simulink library "csbenchlab_sys"  (R2024a)
settings: Solver=VariableStepAuto  StartTime=0.0  StopTime=10.0  RelTol=1e-3
undefined symbols (not defined in the file or in its folder): LinearSystem_data, LinearSystem_DT, LinearSystem_params, LinearSystem_params_merged, LinearSystem_PT, MatlabFunctionSys_data, MatlabFunctionSys_DT, MatlabFunctionSys_params, MatlabFunctionSys_params_merged, MatlabFunctionSys_PT
settings Model: Creator=luka  LastModifiedBy=luka

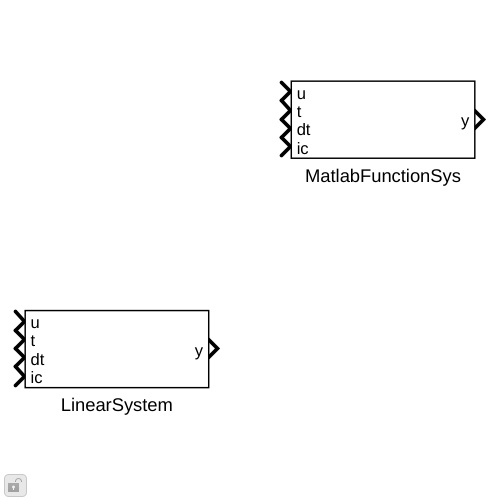
[thumbnail: Simulink's stored preview of the top-level diagram]
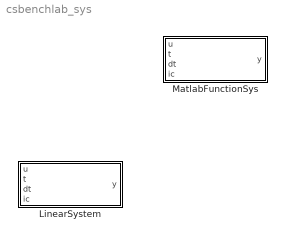
== system csbenchlab_sys ==
  LinearSystem : Subsystem  Tag=__cs_m_sys;  mask{params=LinearSystem_params, params_merged=LinearSystem_params_merged, data=LinearSystem_data, ParamsType=LinearSystem_PT, DataType=LinearSystem_DT}
      mask prompts: params "Parameter struct:"
  MatlabFunctionSys : Subsystem  Tag=__cs_m_sys;  mask{params=MatlabFunctionSys_params, params_merged=MatlabFunctionSys_params_merged, data=MatlabFunctionSys_data, ParamsType=MatlabFunctionSys_PT, DataType=MatlabFunctionSys_DT}
      mask prompts: params "Parameter struct:"

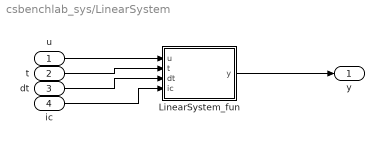
== system csbenchlab_sys/LinearSystem ==
  u : Inport
  t : Inport  Port=2
  dt : Inport  Port=3
  ic : Inport  Port=4
  LinearSystem_fun : MATLAB Function  TreatAsAtomicUnit=on
  y : Outport
  wires:
  u/1 -> LinearSystem_fun/1(u)
  t/1 -> LinearSystem_fun/2(t)
  dt/1 -> LinearSystem_fun/3(dt)
  ic/1 -> LinearSystem_fun/4(ic)
  LinearSystem_fun/1(y) -> y/1

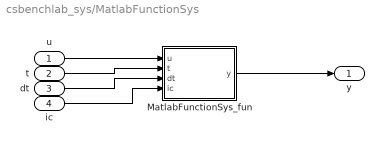
== system csbenchlab_sys/MatlabFunctionSys ==
  u : Inport
  t : Inport  Port=2
  dt : Inport  Port=3
  ic : Inport  Port=4
  MatlabFunctionSys_fun : MATLAB Function  TreatAsAtomicUnit=on
  y : Outport
  wires:
  u/1 -> MatlabFunctionSys_fun/1(u)
  t/1 -> MatlabFunctionSys_fun/2(t)
  dt/1 -> MatlabFunctionSys_fun/3(dt)
  ic/1 -> MatlabFunctionSys_fun/4(ic)
  MatlabFunctionSys_fun/1(y) -> y/1

== matlab function csbenchlab_sys/MatlabFunctionSys/MatlabFunctionSys_fun ==
  settings: updateMethod=DISCRETE
  data: u input; y output; t input; dt input; ic input; data parameter DataType; params parameter ParamsType
% __classname:=MatlabFunctionSys;
function y = fcn(u, t, dt, ic, data, params)
  persistent obj
  if isempty(obj)
    obj = MatlabFunctionSys(params, 'Data', data);
    obj = obj.configure(ic);
  end
 [obj, y] = obj.step(u, t, dt);
end

== matlab function csbenchlab_sys/LinearSystem/LinearSystem_fun ==
  settings: updateMethod=DISCRETE
  data: u input; y output; t input; dt input; ic input; data parameter DataType; params_merged parameter ParamsType
% __classname:=LinearSystem;
function y = fcn(u, t, dt, ic, data, params_merged)
  persistent obj
  if isempty(obj)
    obj = LinearSystem(params, 'Data', data);
    obj = obj.configure(ic);
  end
 [obj, y] = obj.step(u, t, dt);
end
